simulink model "P_Controller"  (R2019a)
settings: Solver=VariableStepAuto  StartTime=0.0  StopTime=10  RelTol=1e-3
undefined symbols (not defined in the file): G1, G2, Kp
settings Model: Creator=Gabe Casciano  LastModifiedBy=Gabe Casciano

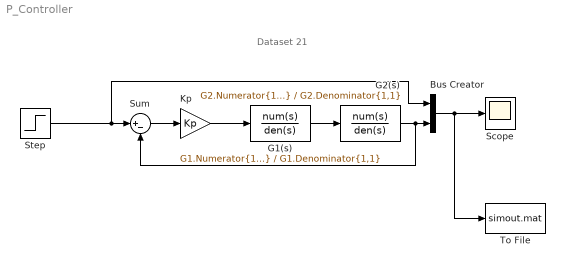
== system P_Controller ==
  note: Dataset 21
  Bus Creator : BusCreator  Inputs=2
  G1(s) : TransferFcn  Numerator=G1.Numerator{1,1}  Denominator=G1.Denominator{1,1}
  G2(s) : TransferFcn  Numerator=G2.Numerator{1,1}  Denominator=G2.Denominator{1,1}
  Kp : Gain  Gain=Kp
  Scope : Scope
  Step : Step  SampleTime=0
  Sum : Sum  Inputs=|+-
  To File : ToFile  Filename=simout.mat  SaveFormat=Timeseries
  wires:
  Bus Creator/1 -> To File/1, Scope/1
  G2(s)/1 -> Sum/2, Bus Creator/2
  G1(s)/1 -> G2(s)/1
  Sum/1 -> Kp/1
  Kp/1 -> G1(s)/1
  Step/1 -> Bus Creator/1, Sum/1
